simulink model "lookup_simu"  (R2019a)
settings: Solver=FixedStepAuto  StartTime=0.0  StopTime=110  FixedStep=10  RelTol=1e-3
values from neighbouring files (symbols this model uses):
  deltaV = 10    [Initialisierung.m]
  ggVLookUp_neg = horzcat(ggVLookUp_neg, interp1(simErg.a_y,simErg.a_x_neg,[0:1:30]'))    [calcggV.m]
  ggVLookUp_pos = horzcat(ggVLookUp_pos, interp1(simErg.a_y,simErg.a_x_pos,[0:1:30]'))    [calcggV.m]
  maxV = 110    [Initialisierung.m]
settings Model: Creator=fried  LastModifiedBy=Frieder Uerlings

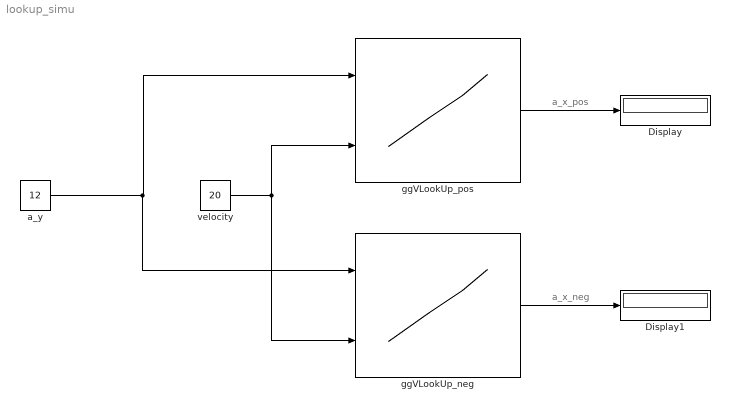
== system lookup_simu ==
  note: a_x_pos
  note: a_x_neg
  Display : Display
  Display1 : Display
  "a_y " : Constant  Value=12
  "ggVLookUp_neg " : Lookup_n-D  BreakpointsForDimension1=[0:1:30]  BreakpointsForDimension2=[0:deltaV:maxV]  Table=ggVLookUp_neg  InternalRulePriority=Speed  RndMeth=Simplest  InputSameDT=on
  "ggVLookUp_pos " : Lookup_n-D  BreakpointsForDimension1=[0:1:30]  BreakpointsForDimension2=[0:deltaV:maxV]  Table=ggVLookUp_pos  InternalRulePriority=Speed  RndMeth=Simplest  InputSameDT=on
  "velocity " : Constant  Value=20
  wires:
  "a_y "/1 -> "ggVLookUp_neg "/1, "ggVLookUp_pos "/1
  "velocity "/1 -> "ggVLookUp_pos "/2, "ggVLookUp_neg "/2
  "ggVLookUp_pos "/1 -> Display/1
  "ggVLookUp_neg "/1 -> Display1/1
